simulink model "TEST_Live_2014"  (Simulink 8.3)
settings: Solver=ode45  SolverMode=SingleTasking  StartTime=0.0  StopTime=10.0  RelTol=1e-3  AbsTol=1e-6
values from neighbouring files (symbols this model uses):
  IFO = 'H1'    [run_NBtest.m]
libraries: cstblocks x3, NbLibrary x3
CloseFcn:
  | ;slview('closediagram',bdroot);
settings Model: Creator=controls  LastModifiedBy=yuta  SimulationMode=external  CovSFcnEnable=on  ExtModeTrigMode=oneshot  ExtModeArmWhenConnect=off
settings DataIOCC: LimitDataPoints=off
settings OptimizationCC: BlockReduction=off  BooleanDataType=off
settings DebuggingCC: SaveWithParameterizedLinksMsg=none  SignalResolutionControl=TryResolveAllWithWarning  SolverPrmCheckMsg=none  MultiTaskDSMMsg=warning  MultiTaskCondExecSysMsg=none  FrameProcessingCompatibilityMsg=error
settings HardwareCC: TargetUnknown=on
settings RTWCC: TemplateMakefile=grt_unix.tmf

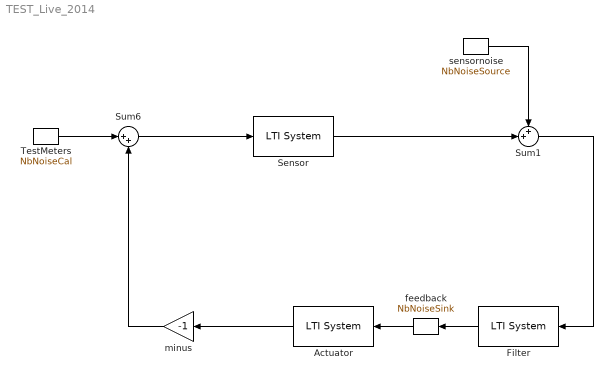
== system TEST_Live_2014 ==
  Actuator : cstblocks/LTI System  sys=Act  IC=[]
  Filter : cstblocks/LTI System  sys=Filt  IC=[]
  Sensor : cstblocks/LTI System  sys=Sen  IC=[]
  Sum1 : Sum  Inputs=++|
  Sum6 : Sum  Inputs=|++
  TestMeters : NbLibrary/NbNoiseCal  Tag=NbNoiseCal  dof='TST'  unit='displacement [m/rtHz]'
      settings: AttributesFormatString=%<Tag>
  feedback : NbLibrary/NbNoiseSink  Tag=NbNoiseSink  dof='TST'  asd=1  chan=[IFO ':LSC-MC_OUT_DQ']
      settings: AttributesFormatString=%<Tag>
  minus : Gain  Gain=-1
  sensornoise : NbLibrary/NbNoiseSource  Tag=NbNoiseSource  asd=1  chan=''  groupNest=1  group='test noise'  subgroup=''  subsubgroup=''  subsubsubgroup=''
      settings: AttributesFormatString=%<Tag>
  wires:
  Actuator/1 -> minus/1
  TestMeters/1 -> Sum6/1
  Sum6/1 -> Sensor/1
  feedback/1 -> Actuator/1
  Filter/1 -> feedback/1
  Sensor/1 -> Sum1/2
  Sum1/1 -> Filter/1
  sensornoise/1 -> Sum1/1
  minus/1 -> Sum6/2
